simulink model "amon_model_EDF"  (R2025b)
settings: Solver=VariableStepAuto  StartTime=0.0  StopTime=T_end  RelTol=1e-3
undefined symbols (not defined in the file): EDF_max, EDF_min, tau_edf
libraries: simulink x1
settings Model: Creator=titit  LastModifiedBy=titit
settings OptimizationCC: DefaultParameterBehavior=Inlined  EnhancedBackFolding=on  PassReuseOutputArgsThreshold=0.0  OptimizeBlockOrder=speed  DifferentSizesBufferReuse=on  OptimizationCustomize=off
settings DebuggingCC: ParameterTunabilityLossMsg=error
settings SFSimCC: MATLABDynamicMemAlloc=off
settings CodeAppCC: ForceParamTrailComments=on  OperatorAnnotations=on

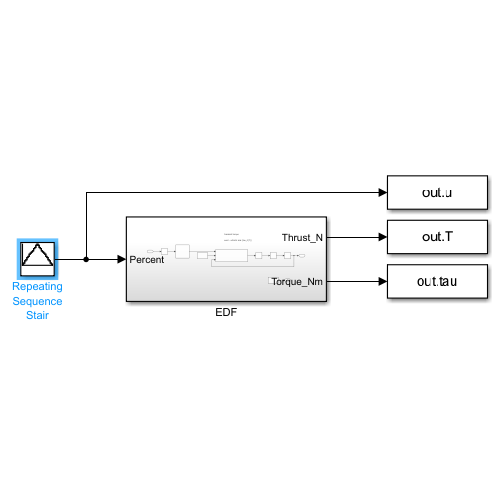
[thumbnail: Simulink's stored preview of the top-level diagram]
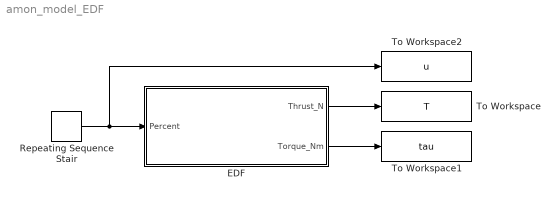
== system amon_model_EDF ==
  EDF : Subsystem
  Repeating Sequence Stair : simulink/Sources/Repeating Sequence Stair  OutValues=EDF_sequence1  tsamp=3  OutMin=[]  OutMax=[]  OutDataTypeStr=double  OutputDataTypeScalingMode=double  OutDataType=fixdt(0,8)  ConRadixGroup=Best Precision: Vector-wise  OutScaling=2^-12
  To Workspace : ToWorkspace  VariableName=T  SaveFormat=Timeseries  SampleTime=-1
  To Workspace1 : ToWorkspace  VariableName=tau  SaveFormat=Timeseries  SampleTime=-1
  To Workspace2 : ToWorkspace  VariableName=u  SaveFormat=Timeseries  SampleTime=-1
  wires:
  EDF/1(Thrust_N) -> To Workspace/1
  EDF/2(Torque_Nm) -> To Workspace1/1
  Repeating Sequence Stair/1 -> To Workspace2/1, EDF/1(Percent)

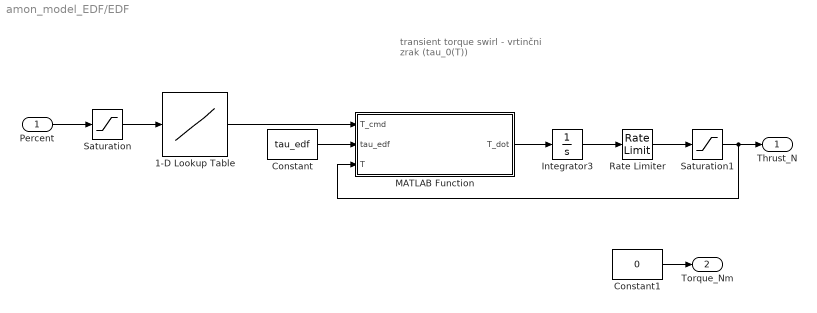
== system amon_model_EDF/EDF ==
  note: transient torque
      | swirl - vrtinčni zrak (tau_0(T))
  Percent : Inport
  1-D Lookup Table : Lookup_n-D  NumberOfTableDimensions=1  BreakpointsForDimension1=[-5:5]  Table=tanh([-5:5])  InternalRulePriority=Speed  RndMeth=Simplest
  Constant : Constant  Value=tau_edf
  Constant1 : Constant  Value=0
  Integrator3 : Integrator
  MATLAB Function : MATLAB Function  TreatAsAtomicUnit=on
  Rate Limiter : RateLimiter  SampleTimeMode=inherited
  Saturation : Saturate  UpperLimit=EDF_max  LowerLimit=EDF_min
  Saturation1 : Saturate  UpperLimit=100  LowerLimit=0
  Thrust_N : Outport
  Torque_Nm : Outport  Port=2
  wires:
  Percent/1 -> Saturation/1
  1-D Lookup Table/1 -> MATLAB Function/1(T_cmd)
  MATLAB Function/1(T_dot) -> Integrator3/1
  Saturation/1 -> 1-D Lookup Table/1
  Constant/1 -> MATLAB Function/2(tau_edf)
  Rate Limiter/1 -> Saturation1/1
  Saturation1/1 -> MATLAB Function/3(T), Thrust_N/1
  Constant1/1 -> Torque_Nm/1
  Integrator3/1 -> Rate Limiter/1

== matlab function amon_model_EDF/EDF/MATLAB Function ==
  data: T_cmd input; tau_edf input; T_dot output; T input
function T_dot = thrust_delay(T_cmd, tau_edf, T)
    T_dot = (1/tau_edf) * (T_cmd - T);
end
